simulink model "boat"  (Simulink 7.9)
settings: Solver=ode45  StartTime=0.0  StopTime=100  RelTol=1e-10
values from neighbouring files (symbols this model uses):
  C = C0    [Minimizer.m]    (also in parameters2.m = [1 0 0 0 0 0;0 0 1 0 0 0;0 0 0 0 1 0]; parameters3.m = [1 0 0 0 0 0;0 0 1 0 0 0;0 0 0 0 1 0])
  fw = 4    [parameters2.m]    (also in parameters3.m)
  I = 1/12*M*((2*rx1)^2 + (2*ry1)^2)    (= 7.46230507536)    [BoatController.m]    (also in boatDynamics.m; parameters2.m = 20; parameters3.m)
  kr = 2    [parameters2.m]    (also in parameters3.m)
  M = 80*lbtokg    (= 36.28736)    [BoatController.m]    (also in parameters2.m = 10; parameters3.m)
libraries: simulink x3
settings Model: Creator=zcc  LastModifiedBy=Darsan
settings GRTTargetCC: CombineOutputUpdateFcns=off  GRTInterface=on

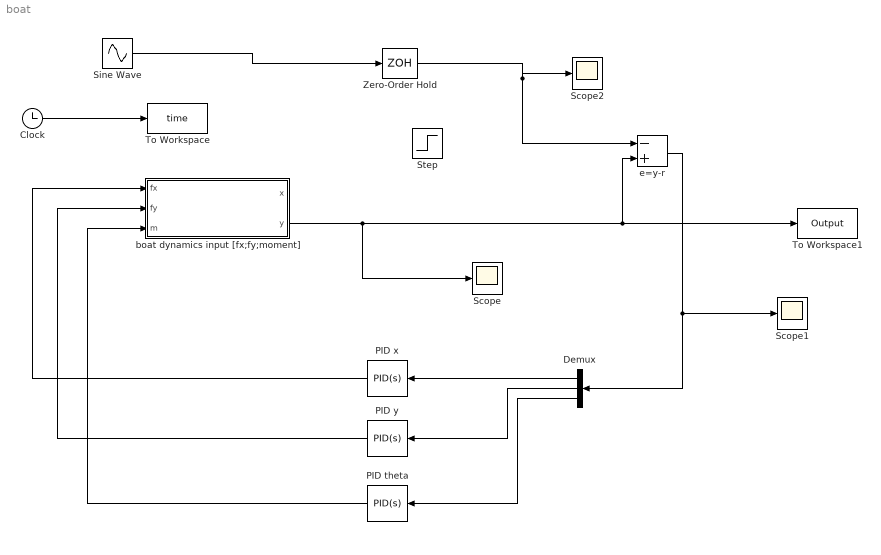
== system boat ==
  Clock : Clock
  Demux : Demux  Outputs=3
  PID theta : simulink/Continuous/PID Controller  Controller=PID  TimeDomain=Continuous-time  SampleTime=1  IntegratorMethod=Forward Euler  FilterMethod=Forward Euler  Form=Parallel  P=-52.7411095906827  I=-178.448916818041  D=5.47077070641916  N=9.64052643054454  InitialConditionSource=internal  InitialConditionForIntegrator=0  InitialConditionForFilter=0  ExternalReset=none  LimitOutput=off  UpperSaturationLimit=inf  LowerSaturationLimit=-inf  LinearizeAsGain=off  AntiWindupMode=none  Kb=1  TrackingMode=off  Kt=1  PParamMin=[]  PParamMax=[]  IParamMin=[]  IParamMax=[]  DParamMin=[]  DParamMax=[]  NParamMin=[]  NParamMax=[]  KbParamMin=[]  KbParamMax=[]  KtParamMin=[]  KtParamMax=[]  POutMin=[]  POutMax=[]  IOutMin=[]  IOutMax=[]  DOutMin=[]  DOutMax=[]  NOutMin=[]  NOutMax=[]  KbOutMin=[]  KbOutMax=[]  KtOutMin=[]  KtOutMax=[]  IntegratorOutMin=[]  IntegratorOutMax=[]  FilterOutMin=[]  FilterOutMax=[]  SumOutMin=[]  SumOutMax=[]  SumI1OutMin=[]  SumI1OutMax=[]  SumI2OutMin=[]  SumI2OutMax=[]  SumI3OutMin=[]  SumI3OutMax=[]  SumDOutMin=[]  SumDOutMax=[]  SaturationOutMin=[]  SaturationOutMax=[]  IntegratorContinuousStateAttributes=''  IntegratorStateMustResolveToSignalObject=off  IntegratorRTWStateStorageClass=Auto  FilterContinuousStateAttributes=''  FilterStateMustResolveToSignalObject=off  FilterRTWStateStorageClass=Auto
  PID x : simulink/Continuous/PID Controller  Controller=PID  TimeDomain=Continuous-time  SampleTime=1  IntegratorMethod=Forward Euler  FilterMethod=Forward Euler  Form=Parallel  P=-52.7411095906827  I=-356.897833636081  D=2.73538535320958  N=19.2810528610891  InitialConditionSource=internal  InitialConditionForIntegrator=0  InitialConditionForFilter=0  ExternalReset=none  LimitOutput=off  UpperSaturationLimit=inf  LowerSaturationLimit=-inf  LinearizeAsGain=off  AntiWindupMode=none  Kb=1  TrackingMode=off  Kt=1  PParamMin=[]  PParamMax=[]  IParamMin=[]  IParamMax=[]  DParamMin=[]  DParamMax=[]  NParamMin=[]  NParamMax=[]  KbParamMin=[]  KbParamMax=[]  KtParamMin=[]  KtParamMax=[]  POutMin=[]  POutMax=[]  IOutMin=[]  IOutMax=[]  DOutMin=[]  DOutMax=[]  NOutMin=[]  NOutMax=[]  KbOutMin=[]  KbOutMax=[]  KtOutMin=[]  KtOutMax=[]  IntegratorOutMin=[]  IntegratorOutMax=[]  FilterOutMin=[]  FilterOutMax=[]  SumOutMin=[]  SumOutMax=[]  SumI1OutMin=[]  SumI1OutMax=[]  SumI2OutMin=[]  SumI2OutMax=[]  SumI3OutMin=[]  SumI3OutMax=[]  SumDOutMin=[]  SumDOutMax=[]  SaturationOutMin=[]  SaturationOutMax=[]  IntegratorContinuousStateAttributes=''  IntegratorStateMustResolveToSignalObject=off  IntegratorRTWStateStorageClass=Auto  FilterContinuousStateAttributes=''  FilterStateMustResolveToSignalObject=off  FilterRTWStateStorageClass=Auto
  PID y : simulink/Continuous/PID Controller  Controller=PID  TimeDomain=Continuous-time  SampleTime=1  IntegratorMethod=Forward Euler  FilterMethod=Forward Euler  Form=Parallel  P=-52.7411095906827  I=-356.897833636081  D=2.73538535320958  N=19.2810528610891  InitialConditionSource=internal  InitialConditionForIntegrator=0  InitialConditionForFilter=0  ExternalReset=none  LimitOutput=off  UpperSaturationLimit=inf  LowerSaturationLimit=-inf  LinearizeAsGain=off  AntiWindupMode=none  Kb=1  TrackingMode=off  Kt=1  PParamMin=[]  PParamMax=[]  IParamMin=[]  IParamMax=[]  DParamMin=[]  DParamMax=[]  NParamMin=[]  NParamMax=[]  KbParamMin=[]  KbParamMax=[]  KtParamMin=[]  KtParamMax=[]  POutMin=[]  POutMax=[]  IOutMin=[]  IOutMax=[]  DOutMin=[]  DOutMax=[]  NOutMin=[]  NOutMax=[]  KbOutMin=[]  KbOutMax=[]  KtOutMin=[]  KtOutMax=[]  IntegratorOutMin=[]  IntegratorOutMax=[]  FilterOutMin=[]  FilterOutMax=[]  SumOutMin=[]  SumOutMax=[]  SumI1OutMin=[]  SumI1OutMax=[]  SumI2OutMin=[]  SumI2OutMax=[]  SumI3OutMin=[]  SumI3OutMax=[]  SumDOutMin=[]  SumDOutMax=[]  SaturationOutMin=[]  SaturationOutMax=[]  IntegratorContinuousStateAttributes=''  IntegratorStateMustResolveToSignalObject=off  IntegratorRTWStateStorageClass=Auto  FilterContinuousStateAttributes=''  FilterStateMustResolveToSignalObject=off  FilterRTWStateStorageClass=Auto
  Scope : Scope
  Scope1 : Scope
      settings: SaveName=ScopeData2
  Scope2 : Scope
      settings: SaveName=ScopeData3
  Sine Wave : Sin  Amplitude=[2;4;700]  Frequency=[2;4;.1]  SampleTime=0
  Step : Step  Before=[0;0;0]  After=[5;2;45]  SampleTime=0
  To Workspace : ToWorkspace  VariableName=time  SampleTime=-1  SaveFormat=Structure
  To Workspace1 : ToWorkspace  VariableName=Output  SampleTime=-1  SaveFormat=Structure
  Zero-Order Hold : ZeroOrderHold  SampleTime=3
  boat dynamics input [fx;fy;moment] : Subsystem  mask{M=M, I=I, fw=fw, kr=kr, C=C}
      mask prompts: M "Mass"; I "Inert"; fw "Water Friction"; kr "Rotational water Friction"; C "Output Matrix"
  e=y-r : Sum  Inputs=-+
  wires:
  boat dynamics input [fx;fy;moment]/2(y) -> Scope/1, e=y-r/2, To Workspace1/1
  e=y-r/1 -> Demux/1, Scope1/1
  Demux/1 -> PID x/1
  Demux/2 -> PID y/1
  Demux/3 -> PID theta/1
  PID x/1 -> boat dynamics input [fx;fy;moment]/1(fx)
  PID y/1 -> boat dynamics input [fx;fy;moment]/2(fy)
  PID theta/1 -> boat dynamics input [fx;fy;moment]/3(m)
  Clock/1 -> To Workspace/1
  Sine Wave/1 -> Zero-Order Hold/1
  Zero-Order Hold/1 -> e=y-r/1, Scope2/1

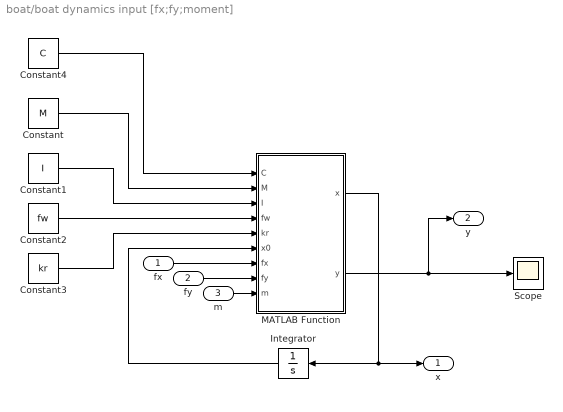
== system boat/boat dynamics input [fx;fy;moment] ==
  fx : Inport
  fy : Inport  Port=2
  m : Inport  Port=3
  Constant : Constant  Value=M
  Constant1 : Constant  Value=I
  Constant2 : Constant  Value=fw
  Constant3 : Constant  Value=kr
  Constant4 : Constant  Value=C
  Integrator : Integrator  InitialCondition=[0 0 0 0 0 0]
  MATLAB Function : MATLAB Function  TreatAsAtomicUnit=on
  Scope : Scope
  x : Outport
  y : Outport  Port=2
  wires:
  MATLAB Function/2(y) -> Scope/1, y/1
  Integrator/1 -> MATLAB Function/6(x0)
  Constant/1 -> MATLAB Function/2(M)
  fx/1 -> MATLAB Function/7(fx)
  Constant1/1 -> MATLAB Function/3(I)
  Constant2/1 -> MATLAB Function/4(fw)
  Constant3/1 -> MATLAB Function/5(kr)
  Constant4/1 -> MATLAB Function/1(C)
  fy/1 -> MATLAB Function/8(fy)
  m/1 -> MATLAB Function/9(m)
  MATLAB Function/1(x) -> Integrator/1, x/1

== matlab function boat dynamics input [fx;fy;moment]/MATLAB Function ==
  data: C input double; x output double; M input double; I input double; fw input double; kr input double; x0 input double; fx input double; y output double; fy input double; m input double
function [x,y] = systemstep(C,M,I,fw,kr,x0,fx,fy,m)

   % status vector y=[x;x_dot;y;_y_dot;theta;theta_dot]
   % forces u=[fx;fy;m]
   % contant parameters {mass; rotational inertia; friction coefficients }
   
   x1 = x0(2);
   x2 = fx/M - x0(2)*fw;
   x3 = x0(4);
   x4 = fy/M - x0(4)*fw;
   x5 = x0(6);
   x6 = m/I - x0(6)*kr;

   x=[x1;x2;x3;x4;x5;x6];
   
   y = C*x;
